simulink model "RTDS_control_test"  (R2022b)
settings: Solver=VariableStepAuto  StartTime=0.0  StopTime=5  RelTol=1e-3
libraries: simulink_extras x1
settings Model: Creator=jackh  LastModifiedBy=jackh

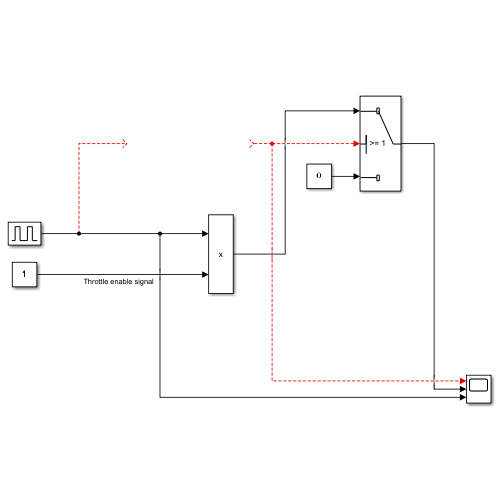
[thumbnail: Simulink's stored preview of the top-level diagram]
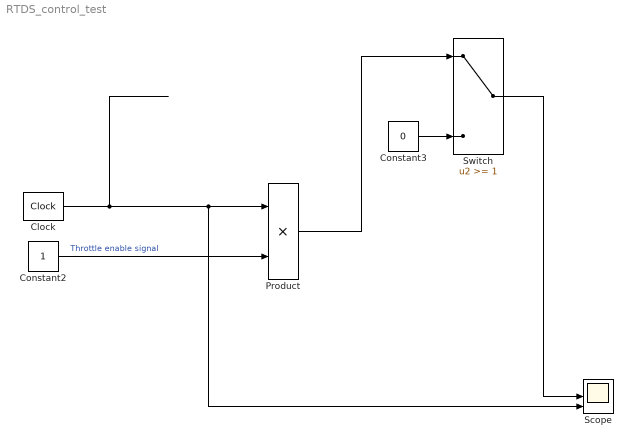
== system RTDS_control_test ==
  Clock : simulink_extras/Flip Flops/Clock  period=1
  Constant2 : Constant
  Constant3 : Constant  Value=0
  Product : Product
  Scope : Scope  NumInputPorts=3
  Switch : Switch  Threshold=1  SaturateOnIntegerOverflow=off  InputSameDT=off
  wires:
  Constant2/1 -> Product/2  "Throttle enable signal"
  Clock/1 -> Scope/3, Product/1
  ? -> Scope/1, Switch/2
  Constant3/1 -> Switch/3
  Product/1 -> Switch/1
  Switch/1 -> Scope/2
